simulink model "Schema_inversione_cinematica_con_inversa_Jacobiano"  (R2023a)
settings: Solver=VariableStepAuto  StartTime=0.0  StopTime=113  RelTol=1e-3
model workspace (MAT data in the model file):
  a = 1
  out_x_error = 1
values from neighbouring files (symbols this model uses):
  a1 = 0.5    [Progetto_FoR.m]
  d0 = 1    [Progetto_FoR.m]
  K = diag(k)    [Progetto_FoR.m]
  q0 = [0 pi/2 0 pi/2]    [Progetto_FoR.m]
  Tc = 0.001    [Progetto_FoR.m]
undefined symbols (not defined in the file or in its folder): DiscIntNeverNeededParam
settings Model: Creator=panto  LastModifiedBy=panto

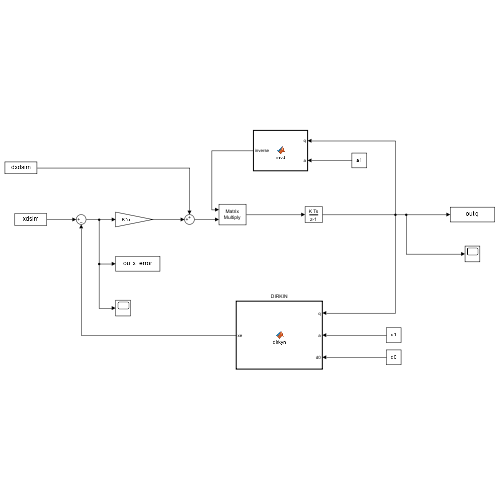
[thumbnail: Simulink's stored preview of the top-level diagram]
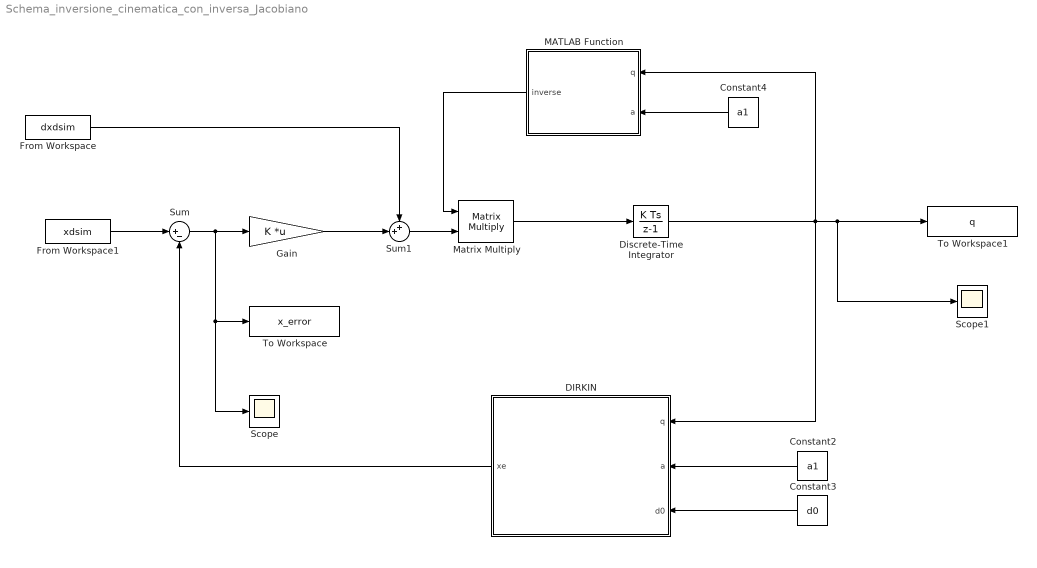
== system Schema_inversione_cinematica_con_inversa_Jacobiano ==
  Constant2 : Constant  Value=a1
  Constant3 : Constant  Value=d0
  Constant4 : Constant  Value=a1
  DIRKIN : MATLAB Function  TreatAsAtomicUnit=on
  Discrete-Time Integrator : DiscreteIntegrator  InitialCondition=q0'  SampleTime=Tc  ICPrevOutput=DiscIntNeverNeededParam  ICPrevScaledInput=DiscIntNeverNeededParam
  From Workspace : FromWorkspace  VariableName=dxdsim  SampleTime=Tc
  From Workspace1 : FromWorkspace  VariableName=xdsim  SampleTime=Tc
  Gain : Gain  Gain=K  Multiplication=Matrix(K*u)
  MATLAB Function : MATLAB Function  TreatAsAtomicUnit=on
  Matrix Multiply : Product  Multiplication=Matrix(*)
  Scope : Scope
  Scope1 : Scope
  Sum : Sum  Inputs=|+-
  Sum1 : Sum  Inputs=++|
  To Workspace : ToWorkspace  VariableName=x_error  SampleTime=Tc
      settings: Save2DSignal=2-D array (concatenate along first dimension)
  To Workspace1 : ToWorkspace  VariableName=q  SampleTime=Tc
      settings: Save2DSignal=2-D array (concatenate along first dimension)
  wires:
  From Workspace1/1 -> Sum/1
  Sum/1 -> To Workspace/1, Scope/1, Gain/1
  From Workspace/1 -> Sum1/1
  Gain/1 -> Sum1/2
  Sum1/1 -> Matrix Multiply/2
  Matrix Multiply/1 -> Discrete-Time Integrator/1
  Discrete-Time Integrator/1 -> Scope1/1, To Workspace1/1, DIRKIN/1(q), MATLAB Function/1(q)
  DIRKIN/1(xe) -> Sum/2
  Constant3/1 -> DIRKIN/3(d0)
  Constant2/1 -> DIRKIN/2(a)
  MATLAB Function/1(inverse) -> Matrix Multiply/1
  Constant4/1 -> MATLAB Function/2(a)

== matlab function Schema_inversione_cinematica_con_inversa_Jacobiano/DIRKIN ==
  data: q input; xe output; a input; d0 input
function xe = dirkyn(q, a, d0)
  xe = zeros(4,1);
    xe = [a*cos(q(1)+q(2))+a*cos(q(1));
        a*sin(q(1)+q(2))+a*sin(q(1));
        d0-q(3);
        q(1)+q(2)-q(4)];
end

== matlab function Schema_inversione_cinematica_con_inversa_Jacobiano/MATLAB Function ==
  data: q input; inverse output; a input
function inverse = invJ(q,a)
%devo prima calcolare lo Jacobiano analitico e poi invertirlo
%Nel caso dello SCARA, lo Jacobiano analitico coincide con quello
%geometrico: questo perchè nello SCARA l'orientamento può essere
%rappresentato direttamente dall'angolo attorno a z, e quindi la velocità
%angolare z si traduce direttamente nella velocità di cambiamento
%dell'angolo di orientamento attorno z
%dal libro when the DOFs cause rotations of the end-effector all about the 
% same fixed axis in space, the two Jacobians are essentially the same
   
    Ja = zeros(4,4);
    Ja = [-a*sin(q(1)+q(2))-a*sin(q(1)) -a*sin(q(1)+q(2)) 0 0;
        a*cos(q(1)+q(2))+a*cos(q(1)) a*cos(q(1)+q(2)) 0 0;
        0 0 -1 0;
        1 1 0 -1];

    inverse = inv(Ja);

end
